simulink model "HexC_FeedbackLinearizationControllerParameterFree"  (R2023a)
settings: Solver=VariableStepAuto  StartTime=0.0  StopTime=tot_time  FixedStep=1e-2  RelTol=1e-3
InitFcn:
  | % INITIALIZATION
  | 
  | A = [zeros(3, 3), eye(3); zeros(3, 6)];
  | 
  | B = [zeros(3, 3); eye(3)];
  | 
  | p = [-2 -2*10 -2*11 -2*12 -2*13 -2*14];
  | 
  | Kv = place(A, B, p);
  | 
  | Kp = Kv(:, 1:3);
  | Kd = Kv(:, 4:6);
  | 
  | p = [-20 -20*10 -20*11 -20*12 -20*13 -20*14];
  | 
  | Ke = place(A, B, p);
  | 
  | sigma = 10;
  | vi = 10;
  | D0 = eye(3)*10;
  | K0 = sigma*D0;
  | 
  | %% UAV PARAMETERS
  | 
  | mass = 1.56779;
  | Ib = diag([0.0347563, 0.0458929, 0.0977]);
  | 
  | %% ESTIMATOR PARAMETERS
  | 
  | syms s;
  | c_0 = 100;
  | poly = (s + c_0)^3;
  | K_est = double(coeffs(poly));
  | 
  | %% PLANNER (ASSUMING THE POINTS IN path HAVE ALREADY BEEN GENERATED WITH RRT)
  | Ts = 1e-3;
  | npoints = length(path(:, 1));
  | tseg = 5;
  | ttot=(npoints-1)*tseg; %duration
  | tdead=10; %dead time to evaluate the steady-state
  | tot_time = ttot + tdead;
  | 
  | t1=linspace(0,tseg,round(tseg/Ts));
  | t=linspace(0,ttot+tdead,round(ttot/Ts)+round(tdead/Ts));
  | 
  | phi_0 = deg2rad(0);
  | theta_0 = deg2rad(0);
  | psi_0 = deg2rad(0);
  | 
  | %p_d= zeros(4,length(t)); dot_p_d= zeros(4,length(t)); ddot_p_d= zeros(4,length(t));
  | p_d = []; dot_p_d = []; ddot_p_d = [];
  | 
  | for i = 1:npoints-1
  |     pi= zeros(6,length(t1)); dot_pi= zeros(6,length(t1)); ddot_pi= zeros(6,length(t1));
  |     %Initial and final conditions
  |     x0= path(i, 1); xf=path(i+1, 1); dot_x0= 0; dot_xf=0; ddot_x0=0; ddot_xf=0; dddot_x0 = 0; dddot_xf = 0;
  |     y0= path(i, 2); yf=path(i+1, 2); dot_y0= 0; dot_yf=0; ddot_y0=0; ddot_yf=0; dddot_y0 = 0; dddot_yf = 0;
  |     z0= path(i, 3); zf=path(i+1, 3); dot_z0= 0; dot_zf=0; ddot_z0=0; ddot_zf=0; dddot_z0 = 0; dddot_zf = 0;
  |     phi0 = phi_0+deg2rad(15*(i-1));
  |     phif=phi_0+deg2rad(15*i); dot_phi0= 0; dot_phif=0; ddot_phi0=0; ddot_phif=0; dddot_phi0 = 0; dddot_phif = 0;
  |     theta0 = theta_0+deg2rad(5*(i-1));
  |     thetaf=theta_0+deg2rad(5*i); dot_theta0= 0; dot_thetaf=0; ddot_theta0=0; ddot_thetaf=0; dddot_theta0 = 0; dddot_thetaf = 0;
  |     psi0 = psi_0+deg2rad(15*(i-1));
  |     psif=psi_0+deg2rad(15*i); dot_psi0= 0; dot_psif=0; ddot_psi0=0; ddot_psif=0; dddot_psi0 = 0; dddot_psif = 0;
  |     p0=[x0,y0,z0,phi0,theta0,psi0]; dot_p0=[dot_x0,dot_y0,dot_z0,dot_phi0,dot_theta0,dot_psi0]; ddot_p0=[ddot_x0,ddot_y0,ddot_z0,ddot_phi0,ddot_theta0,ddot_psi0]; dddot_p0=[dddot_x0,dddot_y0,dddot_z0,dddot_phi0,dddot_theta0,dddot_psi0];
  |     pf=[xf,yf,zf,phif,thetaf,psif]; dot_pf=[dot_xf,dot_yf,dot_zf,dot_phif,dot_thetaf,dot_psif]; ddot_pf=[ddot_xf,ddot_yf,ddot_zf,ddot_phif,ddot_thetaf,ddot_psif]; dddot_pf=[dddot_xf,dddot_yf,dddot_zf,dddot_phif,dddot_thetaf,dddot_psif];
  |     %5-th order polynomial
  |     a0=zeros(1,4); a1=zeros(1,4); a2=zeros(1,4); a3=zeros(1,4); a4=zeros(1,4); a5=zeros(1,4); a6 = zeros(1,4); a7 = zeros(1,4);
  | 
  |     t_iniz = 0;
  |     t_fin = tseg;
  | 
  |     for j=1:6
  |         A = [t_iniz^7, t_iniz^6, t_iniz^5, t_iniz^4, t_iniz^3, t_iniz^2, t_iniz, 1;
  |             t_fin^7, t_fin^6, t_fin^5, t_fin^4, t_fin^3, t_fin^2, t_fin, 1;
  |             7*t_iniz^6, 6*t_iniz^5, 5*t_iniz^4, 4*t_iniz^3, 3*t_iniz^2, 2*t_iniz, 1, 0;
  |             7*t_fin^6, 6*t_fin^5, 5*t_fin^4, 4*t_fin^3, 3*t_fin^2, 2*t_fin, 1, 0;
  |             42*t_iniz^5, 30*t_iniz^4, 20*t_iniz^3, 12*t_iniz^2, 6*t_iniz, 2, 0, 0;
  |             42*t_fin^5, 30*t_fin^4, 20*t_fin^3, 12*t_fin^2, 6*t_fin, 2, 0, 0;
  |             210*t_iniz^4, 120*t_iniz^3, 60*t_iniz^2, 24*t_iniz, 6, 0, 0, 0;
  |             210*t_fin^4, 120*t_fin^3, 60*t_fin^2, 24*t_fin, 6, 0, 0, 0];
  |         b = [p0(j) pf(j) dot_p0(j) dot_pf(j) ddot_p0(j) ddot_pf(j) dddot_p0(j) dddot_pf(j)]';
  |         a_temp = A\b;
  |         a7(j) = a_temp(1);
  |         a6(j) = a_temp(2);
  |         a5(j) = a_temp(3);
  |         a4(j) = a_temp(4);
  |         a3(j) = a_temp(5);
  |         a2(j) = a_temp(6);
  |         a1(j) = a_temp(7);
  |         a0(j) = a_temp(8);
  | 
  |         %trajectories
  |         pi(j,:)=a7(j)*t1.^7 + a6(j)*t1.^6 + a5(j)*t1.^5 +a4(j)*t1.^4 +a3(j)*t1.^3 +a2(j)*t1.^2 +a1(j)*(t1-(i-1)*tseg) +a0(j);
  |         dot_pi(j,:) = 7*a7(j)*t1.^6 + 6*a6(j)*t1.^5 + 5*a5(j)*t1.^4 +4*a4(j)*t1.^3 +3*a3(j)*t1.^2 +2*a2(j)*(t1-(i-1)*tseg) +a1(j);
  |         ddot_pi(j,:) = 42*a7(j)*t1.^5 + 30*a6(j)*t1.^4 + 5*4*a5(j)*t1.^3 +4*3*a4(j)*t1.^2 +3*2*a3(j)*(t1-(i-1)*tseg) +2*a2(j);
  |     end
  | 
  |     % figure(i)
  |     % plot(t1, pi)
  | 
  |     p_d = [p_d pi];
  |     dot_p_d = [dot_p_d dot_pi];
  |     ddot_p_d = [ddot_p_d ddot_pi];
  | 
  | end
  | 
  | %addition of the stead-state terms
  | p_d=[p_d zeros(1,round(tdead/Ts))+p_d(:, end)];
  | dot_p_d=[dot_p_d zeros(1,round(tdead/Ts))+dot_p_d(:, end)];
  | ddot_p_d=[ddot_p_d zeros(1,round(tdead/Ts))+ddot_p_d(:, end)];
  | %data for Simulink
  | pos_0 = [x0 y0 z0];
  | lin_vel_0 = [dot_x0 dot_y0 dot_z0];
  | w_bb_0 = [0 0 0];
  | csi_d=p_d(1:3,:); dot_csi_d=dot_p_d(1:3,:); ddot_csi_d=ddot_p_d(1:3,:);
  | phi_d=p_d(4,:); dot_phi_d=dot_p_d(4,:); ddot_phi_d=ddot_p_d(4,:);
  | theta_d=p_d(5,:); dot_theta_d=dot_p_d(5,:); ddot_theta_d=ddot_p_d(5,:);
  | psi_d=p_d(6,:); dot_psi_d=dot_p_d(6,:); ddot_psi_d=ddot_p_d(6,:);
values from neighbouring files (symbols this model uses):
  i = i+1    (= 1)    [PlannerRRT.m]
  j = j+0.5    (= 0.5)    [PlannerRRT.m]
  path = [path; roadmap(connections(indexPath-2, 2), :)]    [PlannerRRT.m]
undefined symbols (not defined in the file or in its folder): DiscIntNeverNeededParam
libraries: robotcorelib x1, uavutilslib x1
settings Model: Creator=Federico  LastModifiedBy=ricca
settings OptimizationCC: ReuseModelBlockBuffer=off

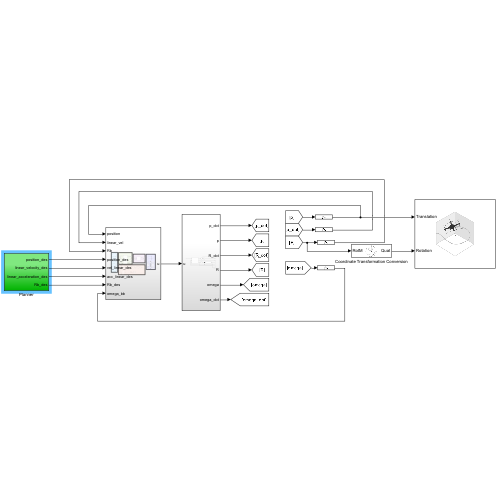
[thumbnail: Simulink's stored preview of the top-level diagram]
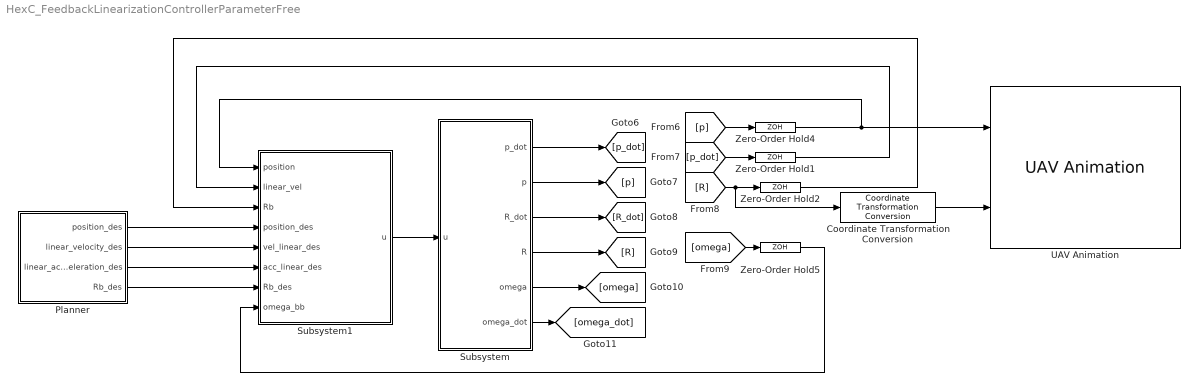
== system HexC_FeedbackLinearizationControllerParameterFree ==
  Coordinate Transformation Conversion : robotcorelib/Coordinate Transformation Conversion  InputRepresentation=Rotation Matrix  InputEulerSequence=ZYX  ShowTrVecInputPort=on  OutputRepresentation=Quaternion  OutputEulerSequence=ZYX  ShowTrVecOutputPort=on  SimulateUsing=Interpreted execution
  Planner : Subsystem
  Subsystem : Subsystem
  Subsystem1 : Subsystem
  UAV Animation : uavutilslib/UAV Animation  UAVType=Multirotor  UAVSize=1  InertialZDirection=Down  SampleTime=0.01
  Zero-Order Hold{1..2,4..5} (4 alike) : ZeroOrderHold  SampleTime=Ts
  wires:
  Subsystem/4(R) -> [R]
  Subsystem/5(omega) -> [omega]
  Subsystem/3(R_dot) -> [R_dot]
  Subsystem/6(omega_dot) -> [omega_dot]
  [p] -> Zero-Order Hold4/1
  [omega] -> Zero-Order Hold5/1
  Subsystem/1(p_dot) -> [p_dot]
  [p_dot] -> Zero-Order Hold1/1
  Zero-Order Hold4/1 -> Subsystem1/1(position), UAV Animation/1
  Coordinate Transformation Conversion/1 -> UAV Animation/2
  [R] -> Coordinate Transformation Conversion/1, Zero-Order Hold2/1
  Subsystem/2(p) -> [p]
  Zero-Order Hold1/1 -> Subsystem1/2(linear_vel)
  Zero-Order Hold2/1 -> Subsystem1/3(Rb)
  Planner/1(position_des) -> Subsystem1/4(position_des)
  Planner/2(linear_velocity_des) -> Subsystem1/5(vel_linear_des)
  Planner/3(linear_acceleration_des) -> Subsystem1/6(acc_linear_des)
  Planner/4(Rb_des) -> Subsystem1/7(Rb_des)
  Subsystem1/1(u) -> Subsystem/1(u)
  Zero-Order Hold5/1 -> Subsystem1/8(omega_bb)

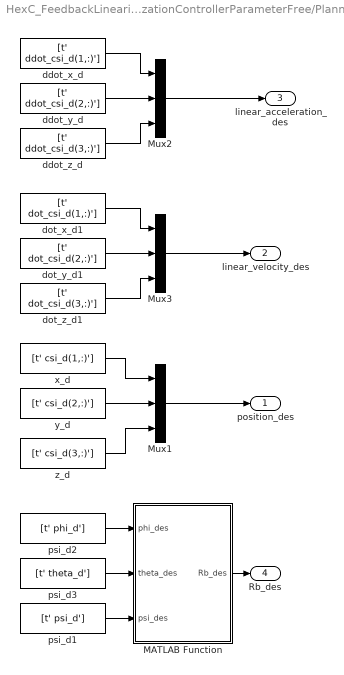
== system HexC_FeedbackLinearizationControllerParameterFree/Planner ==
  MATLAB Function : MATLAB Function  TreatAsAtomicUnit=on
  Mux1 : Mux  Inputs=3
  Mux2 : Mux  Inputs=3
  Mux3 : Mux  Inputs=3
  ddot_x_d : FromWorkspace  VariableName=[t' ddot_csi_d(1,:)']  SampleTime=Ts
  ddot_y_d : FromWorkspace  VariableName=[t' ddot_csi_d(2,:)']  SampleTime=Ts
  ddot_z_d : FromWorkspace  VariableName=[t' ddot_csi_d(3,:)']  SampleTime=Ts
  dot_x_d1 : FromWorkspace  VariableName=[t' dot_csi_d(1,:)']  SampleTime=Ts
  dot_y_d1 : FromWorkspace  VariableName=[t' dot_csi_d(2,:)']  SampleTime=Ts
  dot_z_d1 : FromWorkspace  VariableName=[t' dot_csi_d(3,:)']  SampleTime=Ts
  psi_d1 : FromWorkspace  VariableName=[t' psi_d']  SampleTime=Ts
  psi_d2 : FromWorkspace  VariableName=[t' phi_d']  SampleTime=Ts
  psi_d3 : FromWorkspace  VariableName=[t' theta_d']  SampleTime=Ts
  x_d : FromWorkspace  VariableName=[t' csi_d(1,:)']  SampleTime=Ts
  y_d : FromWorkspace  VariableName=[t' csi_d(2,:)']  SampleTime=Ts
  z_d : FromWorkspace  VariableName=[t' csi_d(3,:)']  SampleTime=Ts
  position_des : Outport
  linear_velocity_des : Outport  Port=2
  linear_acceleration_des : Outport  Port=3
  Rb_des : Outport  Port=4
  wires:
  y_d/1 -> Mux1/2
  z_d/1 -> Mux1/3
  x_d/1 -> Mux1/1
  ddot_y_d/1 -> Mux2/2
  ddot_z_d/1 -> Mux2/3
  ddot_x_d/1 -> Mux2/1
  Mux2/1 -> linear_acceleration_des/1
  Mux1/1 -> position_des/1
  dot_y_d1/1 -> Mux3/2
  dot_z_d1/1 -> Mux3/3
  dot_x_d1/1 -> Mux3/1
  Mux3/1 -> linear_velocity_des/1
  psi_d1/1 -> MATLAB Function/3(psi_des)
  MATLAB Function/1(Rb_des) -> Rb_des/1
  psi_d3/1 -> MATLAB Function/2(theta_des)
  psi_d2/1 -> MATLAB Function/1(phi_des)

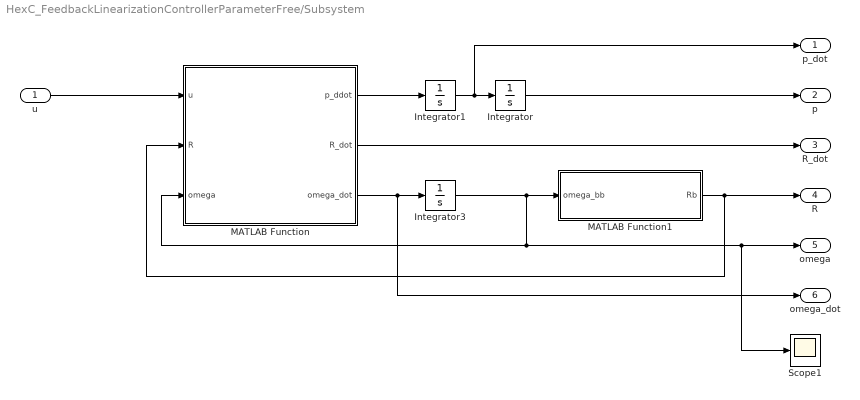
== system HexC_FeedbackLinearizationControllerParameterFree/Subsystem ==
  u : Inport
  Integrator : Integrator  InitialCondition=path(1, :)
  Integrator1 : Integrator
  Integrator3 : Integrator
  MATLAB Function : MATLAB Function  TreatAsAtomicUnit=on
  MATLAB Function1 : MATLAB Function  TreatAsAtomicUnit=on
  Scope1 : Scope
  p_dot : Outport
  p : Outport  Port=2
  R_dot : Outport  Port=3
  R : Outport  Port=4
  omega : Outport  Port=5
  omega_dot : Outport  Port=6
  wires:
  MATLAB Function1/1(Rb) -> MATLAB Function/2(R), R/1
  MATLAB Function/2(R_dot) -> R_dot/1
  MATLAB Function/1(p_ddot) -> Integrator1/1
  Integrator3/1 -> MATLAB Function/3(omega), Scope1/1, omega/1, MATLAB Function1/1(omega_bb)
  Integrator1/1 -> p_dot/1, Integrator/1
  MATLAB Function/3(omega_dot) -> omega_dot/1, Integrator3/1
  Integrator/1 -> p/1
  u/1 -> MATLAB Function/1(u)

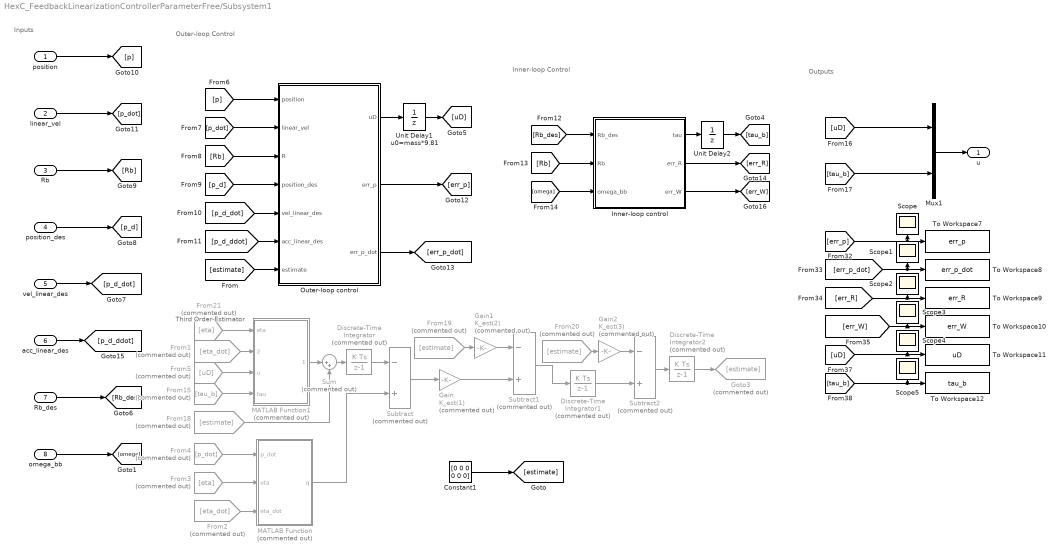
== system HexC_FeedbackLinearizationControllerParameterFree/Subsystem1 ==
  note: Inputs
  note: Outer-loop Control
  note: Inner-loop Control
  note: Outputs
  note: Third Order Estimator
  position : Inport
  linear_vel : Inport  Port=2
  Rb : Inport  Port=3
  position_des : Inport  Port=4
  vel_linear_des : Inport  Port=5
  acc_linear_des : Inport  Port=6
  Rb_des : Inport  Port=7
  omega_bb : Inport  Port=8
  Constant1 : Constant  Value=[0 0 0 0 0 0]
  Discrete-Time Integrator : DiscreteIntegrator  Commented=on  SampleTime=-1  ICPrevOutput=DiscIntNeverNeededParam  ICPrevScaledInput=DiscIntNeverNeededParam
  Discrete-Time Integrator1 : DiscreteIntegrator  Commented=on  SampleTime=-1  ICPrevOutput=DiscIntNeverNeededParam  ICPrevScaledInput=DiscIntNeverNeededParam
  Discrete-Time Integrator2 : DiscreteIntegrator  Commented=on  SampleTime=-1  ICPrevOutput=DiscIntNeverNeededParam  ICPrevScaledInput=DiscIntNeverNeededParam
  From1 : From  Commented=on  GotoTag=eta_dot
  From15 : From  Commented=on  GotoTag=tau_b
  From18 : From  Commented=on  GotoTag=estimate
  From19 : From  Commented=on  GotoTag=estimate
  From2 : From  Commented=on  GotoTag=eta_dot
  From20 : From  Commented=on  GotoTag=estimate
  From21 : From  Commented=on  GotoTag=eta
  From3 : From  Commented=on  GotoTag=eta
  From4 : From  Commented=on  GotoTag=p_dot
  From5 : From  Commented=on  GotoTag=uD
  Gain : Gain  Commented=on  Gain=K_est(1)
  Gain1 : Gain  Commented=on  Gain=K_est(2)
  Gain2 : Gain  Commented=on  Gain=K_est(3)
  Goto3 : Goto  Commented=on  GotoTag=estimate
  Inner-loop control : Subsystem
  MATLAB Function : MATLAB Function  Commented=on  TreatAsAtomicUnit=on
  MATLAB Function1 : MATLAB Function  Commented=on  TreatAsAtomicUnit=on
  Mux1 : Mux  Inputs=2
  Outer-loop control : MATLAB Function  TreatAsAtomicUnit=on
  Scope{,1..5} (6 alike) : Scope
  Subtract : Sum  Commented=on  Inputs=-+
  Subtract1 : Sum  Commented=on  Inputs=-+
  Subtract2 : Sum  Commented=on  Inputs=-+
  Sum : Sum  Commented=on  Inputs=|++
  To Workspace10 : ToWorkspace  VariableName=err_W  SampleTime=-1
  To Workspace11 : ToWorkspace  VariableName=uD  SampleTime=-1
  To Workspace12 : ToWorkspace  VariableName=tau_b  SampleTime=-1
  To Workspace7 : ToWorkspace  VariableName=err_p  SampleTime=-1
  To Workspace8 : ToWorkspace  VariableName=err_p_dot  SampleTime=-1
  To Workspace9 : ToWorkspace  VariableName=err_R  SampleTime=-1
  Unit Delay1 u0=mass*9.81 : UnitDelay  InitialCondition=mass*9.81  SampleTime=Ts
  Unit Delay2 : UnitDelay  InitialCondition=[0 0 0]  SampleTime=Ts
  u : Outport
  wires:
  Unit Delay1 u0=mass*9.81/1 -> [uD]
  Outer-loop control/2(err_p) -> [err_p]
  Outer-loop control/3(err_p_dot) -> [err_p_dot]
  Rb_des/1 -> [Rb_des]
  acc_linear_des/1 -> [p_d_ddot]
  vel_linear_des/1 -> [p_d_dot]
  position_des/1 -> [p_d]
  Rb/1 -> [Rb]
  position/1 -> [p]
  linear_vel/1 -> [p_dot]
  [p] -> Outer-loop control/1(position)
  [p_dot] -> Outer-loop control/2(linear_vel)
  [Rb] -> Outer-loop control/3(R)
  [p_d] -> Outer-loop control/4(position_des)
  [p_d_dot] -> Outer-loop control/5(vel_linear_des)
  [p_d_ddot] -> Outer-loop control/6(acc_linear_des)
  omega_bb/1 -> [omega]
  Outer-loop control/1(uD) -> Unit Delay1 u0=mass*9.81/1
  [Rb_des] -> Inner-loop control/1(Rb_des)
  [Rb] -> Inner-loop control/2(Rb)
  [omega] -> Inner-loop control/3(omega_bb)
  Unit Delay2/1 -> [tau_b]
  Inner-loop control/1(tau) -> Unit Delay2/1
  Inner-loop control/2(err_R) -> [err_R]
  Inner-loop control/3(err_W) -> [err_W]
  [tau_b] -> Mux1/2
  Mux1/1 -> u/1
  [err_p] -> Scope/1, To Workspace7/1
  [err_p_dot] -> To Workspace8/1, Scope1/1
  [err_R] -> Scope2/1, To Workspace9/1
  [tau_b] -> Scope5/1, To Workspace12/1
  [uD] -> Scope4/1, To Workspace11/1
  [err_W] -> Scope3/1, To Workspace10/1
  From18/1 -> Sum/2
  Subtract2/1 -> Discrete-Time Integrator2/1
  From15/1 -> MATLAB Function1/4(tau)
  Gain1/1 -> Subtract1/1
  Discrete-Time Integrator2/1 -> Goto3/1
  From19/1 -> Gain1/1
  Discrete-Time Integrator1/1 -> Subtract2/2
  From4/1 -> MATLAB Function/1(p_dot)
  Sum/1 -> Discrete-Time Integrator/1
  Gain2/1 -> Subtract2/1
  Gain/1 -> Subtract1/2
  From20/1 -> Gain2/1
  MATLAB Function1/1(model_term) -> Sum/1
  From5/1 -> MATLAB Function1/3(u)
  From21/1 -> MATLAB Function1/1(eta)
  Discrete-Time Integrator/1 -> Subtract/1
  MATLAB Function/1(q) -> Subtract/2
  From1/1 -> MATLAB Function1/2(eta_dot)
  From3/1 -> MATLAB Function/2(eta)
  Subtract1/1 -> Discrete-Time Integrator1/1
  From2/1 -> MATLAB Function/3(eta_dot)
  Subtract/1 -> Gain/1
  [estimate] -> Outer-loop control/7(estimate)
  Constant1/1 -> [estimate]
  [uD] -> Mux1/1

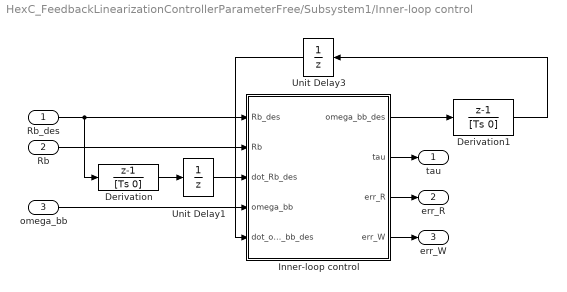
== system HexC_FeedbackLinearizationControllerParameterFree/Subsystem1/Inner-loop control ==
  Rb_des : Inport
  Rb : Inport  Port=2
  omega_bb : Inport  Port=3
  Derivation : DiscreteTransferFcn  Numerator=[1 -1]  Denominator=[Ts 0]  InitialStates=[1 0 0;0 1 0;0 0 1]  SampleTime=Ts
  Derivation1 : DiscreteTransferFcn  Numerator=[1 -1]  Denominator=[Ts 0]  InitialStates=[0 0 0]  SampleTime=Ts
  Inner-loop control : MATLAB Function  TreatAsAtomicUnit=on
  Unit Delay1 : UnitDelay  InitialCondition=eye(3)  SampleTime=Ts
  Unit Delay3 : UnitDelay  InitialCondition=[0 0 0]  SampleTime=Ts
  tau : Outport
  err_R : Outport  Port=2
  err_W : Outport  Port=3
  wires:
  Inner-loop control/3(err_R) -> err_R/1
  Rb/1 -> Inner-loop control/2(Rb)
  Inner-loop control/2(tau) -> tau/1
  Unit Delay1/1 -> Inner-loop control/3(dot_Rb_des)
  Derivation1/1 -> Unit Delay3/1
  Inner-loop control/4(err_W) -> err_W/1
  Unit Delay3/1 -> Inner-loop control/5(dot_omega_bb_des)
  Derivation/1 -> Unit Delay1/1
  Rb_des/1 -> Derivation/1, Inner-loop control/1(Rb_des)
  omega_bb/1 -> Inner-loop control/4(omega_bb)
  Inner-loop control/1(omega_bb_des) -> Derivation1/1

== matlab function HexC_FeedbackLinearizationControllerParameterFree/Planner/MATLAB Function ==
  data: phi_des input; Rb_des output; theta_des input; psi_des input
function Rb_des = fcn(phi_des, theta_des, psi_des)

eta = [phi_des, theta_des, psi_des];

Rb_des = eul2rotm(eta, 'XYZ');

== matlab function HexC_FeedbackLinearizationControllerParameterFree/Subsystem/MATLAB Function1 ==
  data: omega_bb input; Rb output
function Rb = fcn(omega_bb)

    Rb = expm(skew(omega_bb));

end

function S = skew(v)
    if(numel(v)~= 1)
        S= [0 -v(3) v(2); 
            v(3) 0 -v(1);
            -v(2) v(1) 0];
    else
        S= zeros(3);
    end
end

== matlab function HexC_FeedbackLinearizationControllerParameterFree/Subsystem/MATLAB Function ==
  data: u input size=6; R input size=[3,3]; omega input size=3; mass parameter size=1; p_ddot output size=3; R_dot output size=[3,3]; omega_dot output size=3; Ib parameter
% UAV model
function [p_ddot, R_dot, omega_dot] = fcn(u, R, omega, mass, Ib)

    g = 9.81;

    f = u(1:3);
    tau = u(4:6); 

    p_ddot = g*[0;0;1]-1/mass*R*f;
    omega_dot = inv(Ib)*(-skew(omega)*Ib*omega+tau);
    R_dot = R*skew(omega);

end

function S = skew(v)
    if(numel(v)~= 1)
        S= [0 -v(3) v(2); 
            v(3) 0 -v(1);
            -v(2) v(1) 0];
    else
        S= zeros(3);
    end
end

== matlab function HexC_FeedbackLinearizationControllerParameterFree/Subsystem1/Outer-loop control ==
  data: position input size=3; uD output size=3; err_p output size=3; err_p_dot output size=3; linear_vel input size=3; R input size=[3,3]; mass parameter size=1; position_des input size=3; vel_linear_des input size=3; acc_linear_des input size=3; estimate input; Kp parameter; Kd parameter
function [uD, err_p, err_p_dot] = fcn(position, linear_vel, R, mass, position_des, vel_linear_des, acc_linear_des, estimate, Kp, Kd) ...

%% WRITE HERE THE OUTER-LOOP CONTROL

g = 9.81;

err_p = position - position_des;
err_p_dot = linear_vel - vel_linear_des;

uD = inv(R)*mass*([0;0;g]+1/mass*estimate(1:3)+Kp*err_p+Kd*err_p_dot-acc_linear_des);

== matlab function HexC_FeedbackLinearizationControllerParameterFree/Subsystem1/Inner-loop control/Inner-loop control ==
  data: omega_bb_des output size=3; tau output size=3; Rb_des input size=[3,3]; Rb input size=[3,3]; dot_Rb_des input size=[3,3]; omega_bb input size=3; dot_omega_bb_des input size=3; Ib parameter size=[3,3]; err_R output size=3; err_W output size=3
function [omega_bb_des,tau,err_R,err_W] = fcn(Rb_des,Rb,dot_Rb_des,omega_bb,dot_omega_bb_des,Ib)

%% WRITE HERE THE INNER-LOOP CONTROL
% zb_des: desired z-axis of the body frame
% Rb: current rotation matrix
% dot_Rb_des: time-derivative of the desired rotation matrix
% omega_bb: current angular velocity expressed in the body frame
% dot_omega_bb_des: desired angular acceleration expressed in the body
% frame
% xb_des: desired x-axis of the body frame form the planner
% Ib: inertia matrix of the UAV with respect to the body frame
% ---
% Rb_des: desired rotation matrix
% omega_bb_des: desired angular velocity expressed in the body frame (given
% below as a hint)
% tau: commanded control torque
% err_R: rotational error in SO(3)
% err_W: angular velocity error in SO(3)

Kr = 100*eye(3);
Kw = 10*eye(3);

omega_bb_des = wedge(Rb_des'*dot_Rb_des);

err_R = .5*wedge(Rb_des'*Rb-Rb'*Rb_des);
err_W = omega_bb-Rb'*Rb_des*omega_bb_des;
tau = -Kr*err_R-Kw*err_W+skew(omega_bb)*Ib*omega_bb+Ib*(skew(omega_bb)*Rb'*Rb_des*omega_bb_des-Rb'*Rb_des*dot_omega_bb_des);

end

function S = skew(v)
if(numel(v)~= 1)
S= [0 -v(3) v(2); 
    v(3) 0 -v(1);
    -v(2) v(1) 0];
else
S= zeros(3);
end
end

function v = wedge(S)
v1 = S(3,2);
v2 = S(1,3);
v3 = S(2,1);
v = [v1 v2 v3]';
end

== matlab function HexC_FeedbackLinearizationControllerParameterFree/Subsystem1/MATLAB Function ==
  data: p_dot input size=3; q output size=6; eta input size=3; eta_dot input size=3; mass parameter size=1; Ib parameter size=[3,3]
function q = fcn(p_dot, eta, eta_dot, mass, Ib)

    phi = eta(1);
    theta = eta(2);
    psi = eta(3);
    phi_dot = eta_dot(1);
    theta_dot = eta_dot(2);
    psi_dot = eta_dot(3);
    Q = [1 0         -sin(theta);
         0 cos(phi)  cos(theta)*sin(phi);
         0 -sin(phi) cos(theta)*cos(phi)];
    Q_dot = [0 0                 -theta_dot*cos(theta);
             0 -phi_dot*sin(phi) -theta_dot*sin(theta)*sin(phi)+phi_dot*cos(theta)*cos(phi);
             0 -phi_dot*cos(phi) -theta_dot*sin(theta)*cos(phi)-phi_dot*cos(theta)*sin(phi)];
    M = Q'*Ib*Q;
    C = Q'*skew(Q*eta_dot)*Ib*Q+Q'*Ib*Q_dot;
    
    q = [mass*eye(3) zeros(3, 3);
         zeros(3, 3) M]*[p_dot; eta_dot];
    
end

function S = skew(v)
    if(numel(v)~= 1)
        S= [0 -v(3) v(2); 
            v(3) 0 -v(1);
            -v(2) v(1) 0];
    else
        S= zeros(3);
    end
end

== matlab function HexC_FeedbackLinearizationControllerParameterFree/Subsystem1/MATLAB Function1 ==
  data: eta input size=3; eta_dot input size=3; u input size=3; tau input size=3; model_term output size=6; mass parameter size=1; Ib parameter size=[3,3]
function model_term = fcn(eta, eta_dot, u, tau, mass, Ib)

    R = eul2rotm(eta', "XYZ");
    g = 9.81;
    
    phi = eta(1);
    theta = eta(2);
    psi = eta(3);
    phi_dot = eta_dot(1);
    theta_dot = eta_dot(2);
    psi_dot = eta_dot(3);
    Q = [1 0         -sin(theta);
         0 cos(phi)  cos(theta)*sin(phi);
         0 -sin(phi) cos(theta)*cos(phi)];
    Q_dot = [0 0                 -theta_dot*cos(theta);
             0 -phi_dot*sin(phi) -theta_dot*sin(theta)*sin(phi)+phi_dot*cos(theta)*cos(phi);
             0 -phi_dot*cos(phi) -theta_dot*sin(theta)*cos(phi)-phi_dot*cos(theta)*sin(phi)];
    M = Q'*Ib*Q;
    C = Q'*skew(Q*eta_dot)*Ib*Q+Q'*Ib*Q_dot;
    
    model_term = [mass*[0;0;g]-R*u;
        C'*eta_dot+Q'*tau];

end

function S = skew(v)
    if(numel(v)~= 1)
        S= [0 -v(3) v(2); 
            v(3) 0 -v(1);
            -v(2) v(1) 0];
    else
        S= zeros(3);
    end
end
